simulink model "tanks_with_lqr"  (R2017a)
settings: Solver=ode4  StartTime=0.0  StopTime=T  FixedStep=0.001  RelTol=1e-3
values from neighbouring files (symbols this model uses):
  a = 31    [tanks_runner.m]
  b = 40    [tanks_runner.m]
  c = 10    [tanks_runner.m]
  C1 = 16    [tanks_runner.m]
  C2 = 16    [tanks_runner.m]
  C3 = 18    [tanks_runner.m]
  h10 = 20    [tanks_runner.m]
  h20 = 20    [tanks_runner.m]
  h30 = 20    [tanks_runner.m]
  h_max = 40    [tanks_runner.m]
  in_data = [16.0, 15.0, 15.0, 311.75, 100.0, 0, 200.261, 272.519, 52.704, 0.17571237,  0.21817207,  0.07764958]    [setup_experiment.m]    (also in tanks_runner.m = [30.0, 30.0, 22.0, 140.312246999846, 100.0, 0, 128.232384675)
  R = 40    [tanks_runner.m]
  w = 5    [tanks_runner.m]
settings Model: Creator=DUDEKLU  LastModifiedBy=DUDEKLU

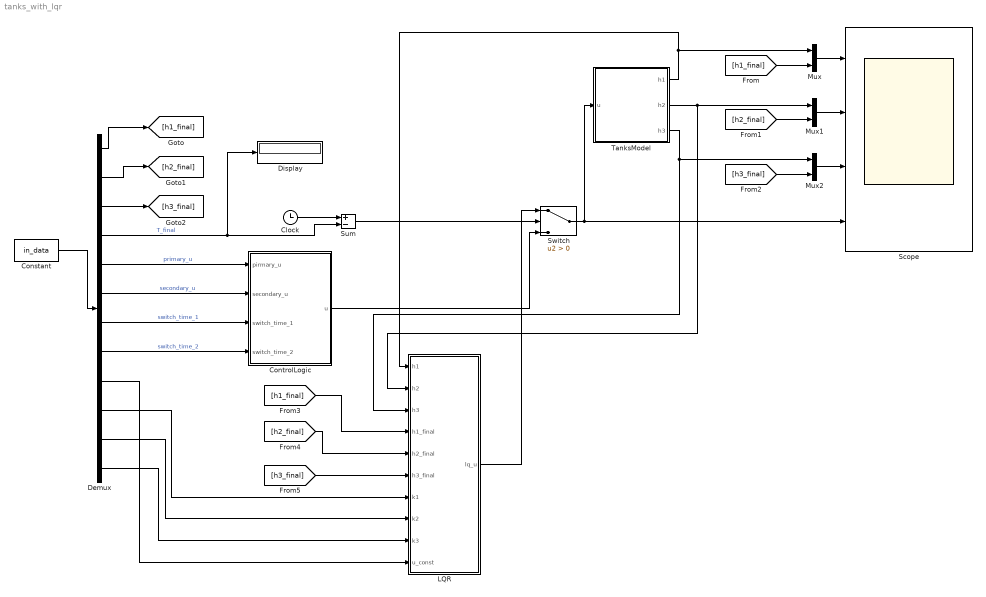
== system tanks_with_lqr ==
  Clock : Clock
  Constant : Constant  Value=in_data
  ControlLogic : Subsystem
  Demux : Demux  Outputs=12
  Display : Display
  LQR : Subsystem
  Mux : Mux  Inputs=2
  Mux1 : Mux  Inputs=2
  Mux2 : Mux  Inputs=2
  Scope : Scope  NumInputPorts=4
  Sum : Sum  Inputs=+-
  Switch : Switch  Criteria=u2 > Threshold
  TanksModel : Subsystem
  wires:
  TanksModel/1(h1) -> LQR/1(h1), Mux/1
  Mux2/1 -> Scope/3
  [h2_final] -> Mux1/2
  Switch/1 -> TanksModel/1(u), Scope/4
  Mux/1 -> Scope/1
  [h3_final] -> Mux2/2
  TanksModel/3(h3) -> Mux2/1, LQR/3(h3)
  [h1_final] -> Mux/2
  Mux1/1 -> Scope/2
  Demux/5 -> ControlLogic/1(pirmary_u)  "primary_u"
  Demux/7 -> ControlLogic/3(switch_time_1)  "switch_time_1"
  Demux/8 -> ControlLogic/4(switch_time_2)  "switch_time_2"
  Demux/1 -> [h1_final]
  Demux/3 -> [h3_final]
  Constant/1 -> Demux/1
  Demux/6 -> ControlLogic/2(secondary_u)  "secondary_u"
  Demux/2 -> [h2_final]
  Demux/4 -> Display/1, Sum/2  "T_final"
  ControlLogic/1(u) -> Switch/3
  LQR/1(lq_u) -> Switch/1
  Clock/1 -> Sum/1
  Sum/1 -> Switch/2
  TanksModel/2(h2) -> LQR/2(h2), Mux1/1
  Demux/9 -> LQR/10(u_const)
  Demux/10 -> LQR/7(k1)
  Demux/11 -> LQR/8(k2)
  Demux/12 -> LQR/9(k3)
  [h1_final] -> LQR/4(h1_final)
  [h2_final] -> LQR/5(h2_final)
  [h3_final] -> LQR/6(h3_final)

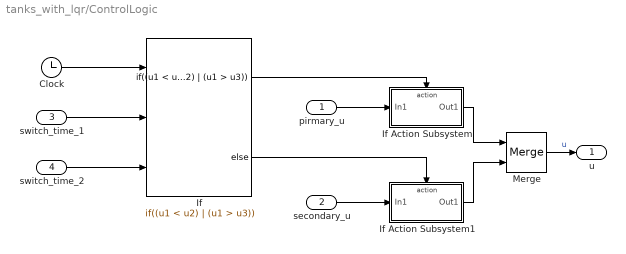
== system tanks_with_lqr/ControlLogic ==
  pirmary_u : Inport
  secondary_u : Inport  Port=2
  switch_time_1 : Inport  Port=3
  switch_time_2 : Inport  Port=4
  Clock : Clock
  If : If  NumInputs=3  IfExpression=(u1 < u2) | (u1 > u3)
  If Action Subsystem : Subsystem  TreatAsAtomicUnit=on
  If Action Subsystem1 : Subsystem  TreatAsAtomicUnit=on
  Merge : Merge
  u : Outport
  wires:
  switch_time_1/1 -> If/2
  secondary_u/1 -> If Action Subsystem1/1(In1)
  switch_time_2/1 -> If/3
  If Action Subsystem1/1(Out1) -> Merge/2
  If/1 -> If Action Subsystem/Action
  If/2 -> If Action Subsystem1/Action
  If Action Subsystem/1(Out1) -> Merge/1
  pirmary_u/1 -> If Action Subsystem/1(In1)
  Clock/1 -> If/1
  Merge/1 -> u/1  "u"

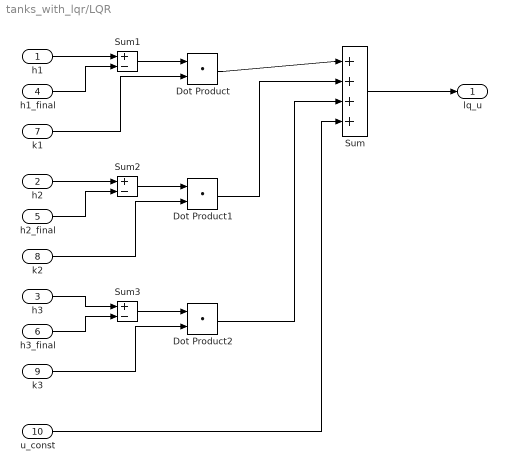
== system tanks_with_lqr/LQR ==
  h1 : Inport
  h2 : Inport  Port=2
  h3 : Inport  Port=3
  h1_final : Inport  Port=4
  h2_final : Inport  Port=5
  h3_final : Inport  Port=6
  k1 : Inport  Port=7
  k2 : Inport  Port=8
  k3 : Inport  Port=9
  u_const : Inport  Port=10
  Dot Product : DotProduct  InputSameDT=on  OutDataTypeStr=Inherit: Inherit via internal rule
  Dot Product1 : DotProduct  InputSameDT=on  OutDataTypeStr=Inherit: Inherit via internal rule
  Dot Product2 : DotProduct  InputSameDT=on  OutDataTypeStr=Inherit: Inherit via internal rule
  Sum : Sum  Inputs=|++++
  Sum1 : Sum  Inputs=+-
  Sum2 : Sum  Inputs=+-
  Sum3 : Sum  Inputs=+-
  lq_u : Outport
  wires:
  h1_final/1 -> Sum1/2
  Sum/1 -> lq_u/1
  h2_final/1 -> Sum2/2
  h3_final/1 -> Sum3/2
  h1/1 -> Sum1/1
  Sum1/1 -> Dot Product/1
  k1/1 -> Dot Product/2
  h2/1 -> Sum2/1
  h3/1 -> Sum3/1
  Sum2/1 -> Dot Product1/1
  k2/1 -> Dot Product1/2
  Sum3/1 -> Dot Product2/1
  k3/1 -> Dot Product2/2
  Dot Product/1 -> Sum/1
  Dot Product1/1 -> Sum/2
  Dot Product2/1 -> Sum/3
  u_const/1 -> Sum/4

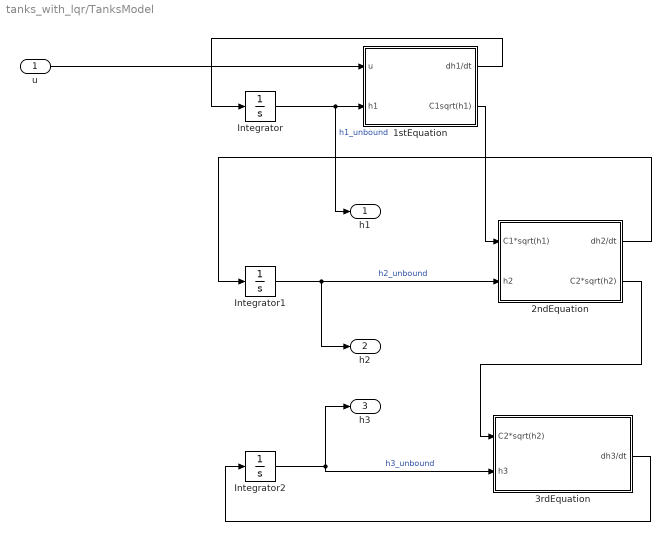
== system tanks_with_lqr/TanksModel ==
  u : Inport
  1stEquation : Subsystem
  2ndEquation : Subsystem
  3rdEquation : Subsystem
  Integrator : Integrator  InitialCondition=h10
  Integrator1 : Integrator  InitialCondition=h20
  Integrator2 : Integrator  InitialCondition=h30
  h1 : Outport
  h2 : Outport  Port=2
  h3 : Outport  Port=3
  wires:
  Integrator1/1 -> 2ndEquation/2(h2), h2/1  "h2_unbound"
  Integrator2/1 -> 3rdEquation/2(h3), h3/1  "h3_unbound"
  Integrator/1 -> h1/1, 1stEquation/2(h1)  "h1_unbound"
  2ndEquation/1(dh2/dt) -> Integrator1/1
  2ndEquation/2(C2*sqrt(h2)) -> 3rdEquation/1(C2*sqrt(h2))
  3rdEquation/1(dh3/dt) -> Integrator2/1
  1stEquation/1(dh1/dt) -> Integrator/1
  1stEquation/2(C1sqrt(h1)) -> 2ndEquation/1(C1*sqrt(h1))
  u/1 -> 1stEquation/1(u)

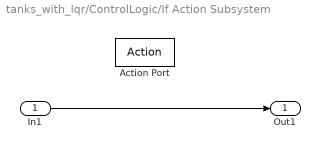
== system tanks_with_lqr/ControlLogic/If Action Subsystem ==
  In1 : Inport
  Action Port : ActionPort  ActionType=then
  Out1 : Outport
  wires:
  In1/1 -> Out1/1

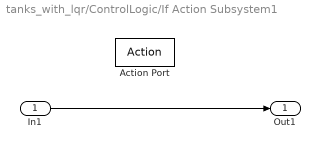
== system tanks_with_lqr/ControlLogic/If Action Subsystem1 ==
  In1 : Inport
  Action Port : ActionPort  ActionType=else
  Out1 : Outport
  wires:
  In1/1 -> Out1/1

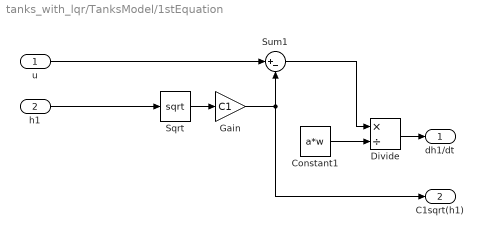
== system tanks_with_lqr/TanksModel/1stEquation ==
  u : Inport
  h1 : Inport  Port=2
  Constant1 : Constant  Value=a*w
  Divide : Product  Inputs=*/
  Gain : Gain  Gain=C1
  Sqrt : Sqrt  SaturateOnIntegerOverflow=on
  Sum1 : Sum  Inputs=|+-
  dh1/dt : Outport
  C1sqrt(h1) : Outport  Port=2
  wires:
  h1/1 -> Sqrt/1
  Constant1/1 -> Divide/2
  Divide/1 -> dh1/dt/1
  u/1 -> Sum1/1
  Gain/1 -> C1sqrt(h1)/1, Sum1/2
  Sqrt/1 -> Gain/1
  Sum1/1 -> Divide/1

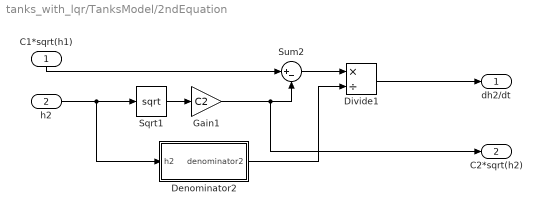
== system tanks_with_lqr/TanksModel/2ndEquation ==
  C1*sqrt(h1) : Inport
  h2 : Inport  Port=2
  Denominator2 : Subsystem
  Divide1 : Product  Inputs=*/
  Gain1 : Gain  Gain=C2
  Sqrt1 : Sqrt  SaturateOnIntegerOverflow=on
  Sum2 : Sum  Inputs=|+-
  dh2/dt : Outport
  C2*sqrt(h2) : Outport  Port=2
  wires:
  Sqrt1/1 -> Gain1/1
  Gain1/1 -> C2*sqrt(h2)/1, Sum2/2
  Denominator2/1(denominator2) -> Divide1/2
  Sum2/1 -> Divide1/1
  h2/1 -> Denominator2/1(h2), Sqrt1/1
  C1*sqrt(h1)/1 -> Sum2/1
  Divide1/1 -> dh2/dt/1

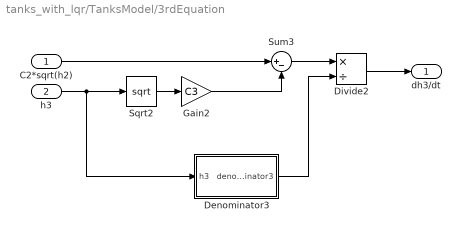
== system tanks_with_lqr/TanksModel/3rdEquation ==
  C2*sqrt(h2) : Inport
  h3 : Inport  Port=2
  Denominator3 : Subsystem
  Divide2 : Product  Inputs=*/
  Gain2 : Gain  Gain=C3
  Sqrt2 : Sqrt  SaturateOnIntegerOverflow=on
  Sum3 : Sum  Inputs=|+-
  dh3/dt : Outport
  wires:
  Sum3/1 -> Divide2/1
  Divide2/1 -> dh3/dt/1
  Sqrt2/1 -> Gain2/1
  Gain2/1 -> Sum3/2
  Denominator3/1(denominator3) -> Divide2/2
  C2*sqrt(h2)/1 -> Sum3/1
  h3/1 -> Denominator3/1(h3), Sqrt2/1

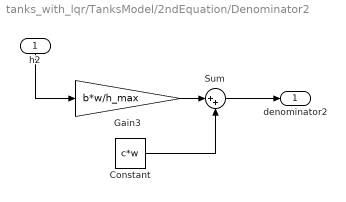
== system tanks_with_lqr/TanksModel/2ndEquation/Denominator2 ==
  h2 : Inport
  Constant : Constant  Value=c*w
  Gain3 : Gain  Gain=b*w/h_max
  Sum : Sum  Inputs=|++
  denominator2 : Outport
  wires:
  Sum/1 -> denominator2/1
  Constant/1 -> Sum/2
  h2/1 -> Gain3/1
  Gain3/1 -> Sum/1

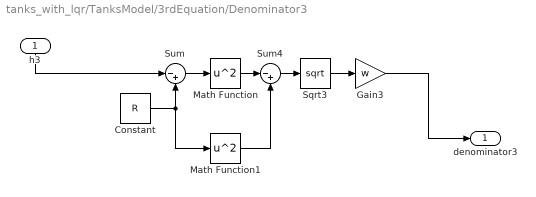
== system tanks_with_lqr/TanksModel/3rdEquation/Denominator3 ==
  h3 : Inport
  Constant : Constant  Value=R
  Gain3 : Gain  Gain=w
  Math Function : Math  Operator=square  SaturateOnIntegerOverflow=on
  Math Function1 : Math  Operator=square  SaturateOnIntegerOverflow=on
  Sqrt3 : Sqrt  SaturateOnIntegerOverflow=on
  Sum : Sum  Inputs=|-+
  Sum4 : Sum  Inputs=|-+
  denominator3 : Outport
  wires:
  Sum/1 -> Math Function/1
  Sqrt3/1 -> Gain3/1
  Math Function1/1 -> Sum4/2
  Sum4/1 -> Sqrt3/1
  h3/1 -> Sum/1
  Math Function/1 -> Sum4/1
  Gain3/1 -> denominator3/1
  Constant/1 -> Sum/2, Math Function1/1
